simulink model "mppt"  (R2025b)
settings: Solver=VariableStepAuto  StartTime=0.0  StopTime=3  RelTol=1e-3
undefined symbols (not defined in the file): magnitude
libraries: spsParallelRLCBranchLib x8, spsVoltageMeasurementLib x3, spsCurrentMeasurementLib x2, spsDiodeLib x2, spsIGBTDiodeLib x2, spsPVArrayLib x2, eePwmGenerator x2, sps_lib x1, spspowerguiLib x1
settings Model: Creator=周宇轩  LastModifiedBy=yuxuan
settings SolverCC: ZeroCrossAlgorithm=Adaptive
settings DataIOCC: Refine=10
settings DebuggingCC: MaskedZcDiagnostic=none  IgnoredZcDiagnostic=none
settings RTWCC: GPUComputeCapability=3.5

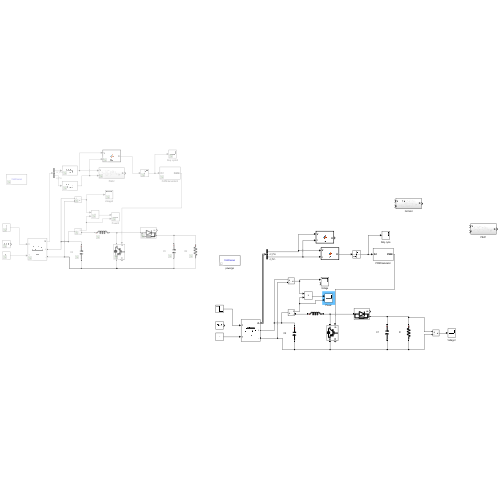
[thumbnail: Simulink's stored preview of the top-level diagram]
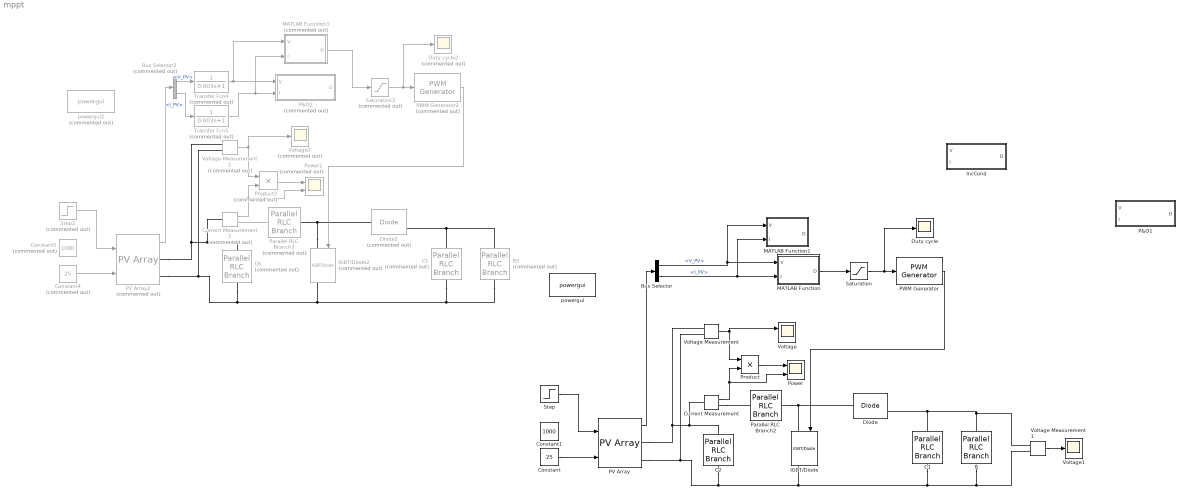
== system mppt ==
  Bus Selector : BusSelector  OutputSignals=V_PV,I_PV
  Bus Selector2 : BusSelector  Commented=on  OutputSignals=V_PV,I_PV
  C1 : spsParallelRLCBranchLib/Parallel RLC Branch  LConnTagsString=a  RConnTagsString=__new0  BranchType=C  Resistance=0  Inductance=0  SetiL0=off  InitialCurrent=0  Capacitance=1e-3  Setx0=off  InitialVoltage=0  Measurements=None
  C2 : spsParallelRLCBranchLib/Parallel RLC Branch  LConnTagsString=a  RConnTagsString=__new0  BranchType=C  Resistance=0  Inductance=0  SetiL0=off  InitialCurrent=0  Capacitance=2e-3  Setx0=off  InitialVoltage=0  Measurements=None
  C5 : spsParallelRLCBranchLib/Parallel RLC Branch  Commented=on  LConnTagsString=a  RConnTagsString=__new0  BranchType=C  Resistance=0  Inductance=0  SetiL0=off  InitialCurrent=0  Capacitance=1e-3  Setx0=off  InitialVoltage=0  Measurements=None
  C6 : spsParallelRLCBranchLib/Parallel RLC Branch  Commented=on  LConnTagsString=a  RConnTagsString=__new0  BranchType=C  Resistance=0  Inductance=0  SetiL0=off  InitialCurrent=0  Capacitance=1e-3  Setx0=off  InitialVoltage=0  Measurements=None
  Constant : Constant  Value=25
  Constant1 : Constant  Value=1000
  Constant4 : Constant  Commented=on  Value=25
  Constant5 : Constant  Commented=on  Value=1000
  Current Measurement : spsCurrentMeasurementLib/Current Measurement  PhasorSimulation=off  OutputType=Complex  PSBequivalent=0
  Current Measurement2 : spsCurrentMeasurementLib/Current Measurement  Commented=on  PhasorSimulation=off  OutputType=Complex  PSBequivalent=0
  Diode : spsDiodeLib/Diode  Ron=0.001  Lon=0  Vf=0.8  IC=0  UseSnubber=0  Rs=500  Cs=250e-9  Measurements=on
  Diode2 : spsDiodeLib/Diode  Commented=on  Ron=0.001  Lon=0  Vf=0.8  IC=0  UseSnubber=0  Rs=500  Cs=250e-9  Measurements=on
  Duty cycle : Scope
      settings: ActiveDisplayYMinimum=-0.03987  ActiveDisplayYMaximum=0.35887
  Duty cycle2 : Scope  Commented=on
      settings: ActiveDisplayYMinimum=-0.03987  ActiveDisplayYMaximum=0.35887  DataLoggingVariableName=ScopeData4
  IGBT/Diode : spsIGBTDiodeLib/IGBT//Diode  Ron=1e-3  Rs=1e5  Cs=inf  Measurements=on
  IGBT/Diode2 : spsIGBTDiodeLib/IGBT//Diode  Commented=on  Ron=1e-3  Rs=1e5  Cs=inf  Measurements=on
  IncCond : Subsystem
  MATLAB Function : MATLAB Function  TreatAsAtomicUnit=on
  MATLAB Function1 : MATLAB Function  TreatAsAtomicUnit=on
  MATLAB Function3 : MATLAB Function  Commented=on  TreatAsAtomicUnit=on
  P&O1 : Subsystem
  P&O2 : Subsystem  Commented=on
  PV Array : spsPVArrayLib/PV Array  Npar=40  Nser=10  PlotType=array @ 25 deg.C & specified irradiances  S_vec="[ 1000  600  100 ]"  Temp_C_vec="[ 45 25  ]"  ModuleName=User-defined  PlotWhenSelected=off  Pm=213.15  Ncell=60  Voc=36.3  Isc=7.84  Vm=29  Im=7.35  beta_Voc_pc=-0.36099  alpha_Isc_pc=0.102  beta_Voc=-0.13104  alpha_Isc=0.0079968  IL=7.8654  I0=2.9273e-10  nI=0.98119  Rsh=313.0553  Rs=0.39381  RobustModel=off  RobustCellTemperature=313.3991  BAL=on  Tc=1e-6  Tfilter=5e-5
  PV Array2 : spsPVArrayLib/PV Array  Commented=on  Npar=40  Nser=10  PlotType=array @ 25 deg.C & specified irradiances  S_vec="[ 1000  600  100 ]"  Temp_C_vec="[ 45 25  ]"  ModuleName=User-defined  PlotWhenSelected=off  Pm=213.15  Ncell=60  Voc=36.3  Isc=7.84  Vm=29  Im=7.35  beta_Voc_pc=-0.36099  alpha_Isc_pc=0.102  beta_Voc=-0.13104  alpha_Isc=0.0079968  IL=7.8654  I0=2.9273e-10  nI=0.98119  Rsh=313.0553  Rs=0.39381  RobustModel=off  RobustCellTemperature=313.3991  BAL=on  Tc=1e-6  Tfilter=5e-5
  PWM Generator : eePwmGenerator/PWM Generator  CarrCount=Up  Tper=0.0001  Tdelay=0  Ts=5e-6
  PWM Generator2 : eePwmGenerator/PWM Generator  Commented=on  CarrCount=Up  Tper=0.001  Tdelay=0  Ts=5e-5
  Parallel RLC Branch2 : spsParallelRLCBranchLib/Parallel RLC Branch  LConnTagsString=a  RConnTagsString=__new0  BranchType=L  Resistance=0  Inductance=3e-3  SetiL0=off  InitialCurrent=0  Capacitance=0  Setx0=off  InitialVoltage=0  Measurements=None
  Parallel RLC Branch3 : spsParallelRLCBranchLib/Parallel RLC Branch  Commented=on  LConnTagsString=a  RConnTagsString=__new0  BranchType=L  Resistance=0  Inductance=1e-3  SetiL0=off  InitialCurrent=0  Capacitance=0  Setx0=off  InitialVoltage=0  Measurements=None
  Power : Scope  NumInputPorts=2
      settings: ActiveDisplayYMinimum=-12032.8561078076  ActiveDisplayYMaximum=108295.70497026842
  Power2 : Scope  Commented=on  NumInputPorts=2
      settings: ActiveDisplayYMinimum=12927.91073  ActiveDisplayYMaximum=92933.50391  DataLoggingVariableName=ScopeData5
  Product : Product
  Product2 : Product  Commented=on
  R : spsParallelRLCBranchLib/Parallel RLC Branch  LConnTagsString=a  RConnTagsString=__new0  BranchType=R  Resistance=2  Inductance=0  SetiL0=off  InitialCurrent=0  Capacitance=0  Setx0=off  InitialVoltage=0  Measurements=None
  R2 : spsParallelRLCBranchLib/Parallel RLC Branch  Commented=on  LConnTagsString=a  RConnTagsString=__new0  BranchType=R  Resistance=2  Inductance=0  SetiL0=off  InitialCurrent=0  Capacitance=0  Setx0=off  InitialVoltage=0  Measurements=None
  Saturation : Saturate  UpperLimit=0.95  LowerLimit=0.05
  Saturation2 : Saturate  Commented=on  UpperLimit=0.95  LowerLimit=0.05
  Step : Step  Time=0.5  Before=1e3  After=600  SampleTime=0
  Step2 : Step  Commented=on  Time=0.5  Before=1e3  After=600  SampleTime=0
  Transfer Fcn4 : TransferFcn  Commented=on  Denominator=[0.003 1]
  Transfer Fcn5 : TransferFcn  Commented=on  Denominator=[0.003 1]
  Voltage : Scope  NumInputPorts=2
      settings: MaximizeAxes=On  ActiveDisplayYMinimum=-41.254198006758806  ActiveDisplayYMaximum=371.28778206082933
  Voltage Measurement : spsVoltageMeasurementLib/Voltage Measurement  PhasorSimulation=off  OutputType=Complex  PSBequivalent=0
  Voltage Measurement1 : spsVoltageMeasurementLib/Voltage Measurement  PhasorSimulation=off  OutputType=Complex  PSBequivalent=0
  Voltage Measurement2 : spsVoltageMeasurementLib/Voltage Measurement  Commented=on  PhasorSimulation=off  OutputType=Complex  PSBequivalent=0
  Voltage1 : Scope
      settings: MaximizeAxes=On  ActiveDisplayYMinimum=-41.254198006758806  ActiveDisplayYMaximum=371.28778206082933  DataLoggingVariableName=ScopeData2
  Voltage2 : Scope  Commented=on
      settings: MaximizeAxes=On  ActiveDisplayYMinimum=-213.56323  ActiveDisplayYMaximum=413.80386  DataLoggingVariableName=ScopeData6
  powergui : sps_lib/powergui  Priority=1  SimulationMode=Continuous  SampleTime=50e-6  frequency=60  Iterations=50  frequencyindice=0  Pbase=100e6  ErrMax=1e-4  UnitsV=kV  UnitsW=MW  buscounter=0  FunctionMessages=off  echomessages=off  EnableUseOfTLC=off  CurrentSourceSwitches=off  DisableSnubberDevices=off  DisableRonSwitches=off  DisableVfSwitches=off  DisplayEquations=off  AutomaticDiscreteSolvers=off  SolverType=Tustin/Backward Euler (TBE)  Interpol=off  ExternalGateDelay=off  methode=off  Ts=100  x0status=blocks  SPID=on  SwTol=0  HookPort=off  NonlinearTolerance=1e-4  nMaxIteration=100  ContinueOnMaxIteration=off  RestoreLinks=warning  ResistiveCurrentMeasurement=off  Frange=[0:2:500]  Ylog=off  Xlog=on  ShowGrid=off  save=off  variable=ZData  structure=0  ZoomFFT=off  StartTime=0.0  cycles=1  DisplayStyle=1  fundamental=60  FreqAxis=off  MaxFrequency=1000  frequencyindicesteady=1  RmsSteady=1  display=off
  powergui2 : spspowerguiLib/powergui  Priority=1  Commented=on  SimulationMode=Continuous  SampleTime=50e-6  frequency=60  Iterations=50  frequencyindice=0  Pbase=100e6  ErrMax=1e-4  UnitsV=kV  UnitsW=MW  buscounter=0  FunctionMessages=off  echomessages=off  EnableUseOfTLC=off  CurrentSourceSwitches=off  DisableSnubberDevices=off  DisableRonSwitches=off  DisableVfSwitches=off  DisplayEquations=off  AutomaticDiscreteSolvers=off  SolverType=Tustin/Backward Euler (TBE)  Interpol=off  ExternalGateDelay=off  methode=off  Ts=100  x0status=blocks  SPID=on  SwTol=0  HookPort=off  NonlinearTolerance=1e-4  nMaxIteration=100  ContinueOnMaxIteration=off  RestoreLinks=warning  ResistiveCurrentMeasurement=off  Frange=[0:2:500]  Ylog=off  Xlog=on  ShowGrid=off  save=off  variable=ZData  structure=0  ZoomFFT=off  StartTime=0.0  cycles=1  DisplayStyle=1  fundamental=60  FreqAxis=off  MaxFrequency=1000  frequencyindicesteady=1  RmsSteady=1  display=off
  wires:
  Constant/1 -> PV Array/2
  Bus Selector/1 -> MATLAB Function1/1(V), MATLAB Function/1(V)  "<V_PV>"
  Bus Selector/2 -> MATLAB Function1/2(I), MATLAB Function/2(I)  "<I_PV>"
  PV Array/1 -> Bus Selector/1
  Current Measurement/1 -> Power/2, Product/2
  Product/1 -> Power/1
  Voltage Measurement/1 -> Voltage/1, Product/1
  PWM Generator/1 -> IGBT/Diode/1
  Saturation/1 -> Duty cycle/1, PWM Generator/1
  Current Measurement2/1 -> Power2/2, Product2/2
  Saturation2/1 -> Duty cycle2/1, PWM Generator2/1
  Product2/1 -> Power2/1
  MATLAB Function3/1(D) -> Saturation2/1
  Voltage Measurement2/1 -> Voltage2/1, Product2/1
  PWM Generator2/1 -> IGBT/Diode2/1
  Constant4/1 -> PV Array2/2
  Bus Selector2/1 -> Transfer Fcn4/1  "<V_PV>"
  Bus Selector2/2 -> Transfer Fcn5/1  "<I_PV>"
  Step2/1 -> PV Array2/1
  Transfer Fcn4/1 -> P&O2/1(V), MATLAB Function3/1(V)
  Transfer Fcn5/1 -> P&O2/2(I), MATLAB Function3/2(I)
  PV Array2/1 -> Bus Selector2/1
  Step/1 -> PV Array/1
  MATLAB Function/1(D) -> Saturation/1
  Voltage Measurement1/1 -> Voltage1/1
  connections:
  Diode/LConn1 -- Parallel RLC Branch2/RConn1 -- IGBT/Diode/LConn1
  PV Array/RConn2 -- Voltage Measurement/LConn2 -- R/RConn1 -- Voltage Measurement1/LConn2 -- C1/RConn1 -- IGBT/Diode/RConn1 -- C2/RConn1
  R/LConn1 -- Voltage Measurement1/LConn1 -- C1/LConn1 -- Diode/RConn1
  PV Array/RConn1 -- Voltage Measurement/LConn1 -- Current Measurement/LConn1 -- C2/LConn1
  Current Measurement/RConn1 -- Parallel RLC Branch2/LConn1
  IGBT/Diode2/RConn1 -- PV Array2/RConn2 -- Voltage Measurement2/LConn2 -- C6/RConn1 -- R2/RConn1 -- C5/RConn1
  C6/LConn1 -- PV Array2/RConn1 -- Voltage Measurement2/LConn1 -- Current Measurement2/LConn1
  Diode2/RConn1 -- R2/LConn1 -- C5/LConn1
  IGBT/Diode2/LConn1 -- Diode2/LConn1 -- Parallel RLC Branch3/RConn1
  Current Measurement2/RConn1 -- Parallel RLC Branch3/LConn1

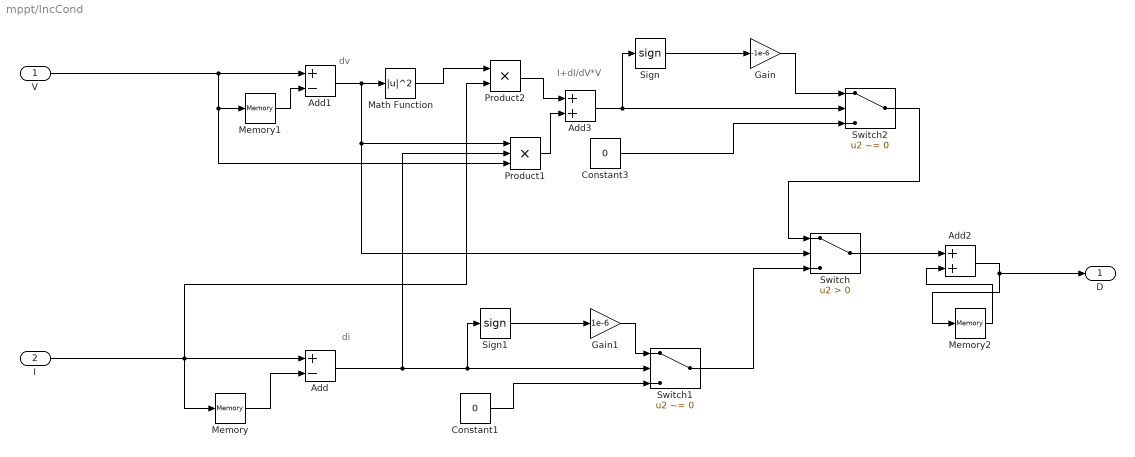
== system mppt/IncCond ==
  note: I+dI/dV*V
  note: di
  note: dv
  V : Inport
  I : Inport  Port=2
  Add : Sum  Inputs=+-
  Add1 : Sum  Inputs=+-
  Add2 : Sum
  Add3 : Sum
  Constant1 : Constant  Value=0
  Constant3 : Constant  Value=0
  Gain : Gain  Gain=-1e-6
  Gain1 : Gain  Gain=1e-6
  Math Function : Math  Operator=magnitude^2
  Memory : Memory
  Memory1 : Memory
  Memory2 : Memory
  Product1 : Product  Inputs=3
  Product2 : Product
  Sign : Signum
  Sign1 : Signum
  Switch : Switch  Criteria=u2 > Threshold  SaturateOnIntegerOverflow=off  InputSameDT=off
  Switch1 : Switch  Criteria=u2 ~= 0  SaturateOnIntegerOverflow=off  InputSameDT=off
  Switch2 : Switch  Criteria=u2 ~= 0  SaturateOnIntegerOverflow=off  InputSameDT=off
  D : Outport
  wires:
  Memory/1 -> Add/2
  V/1 -> Product1/3, Memory1/1, Add1/1
  Add1/1 -> Switch/2, Product1/1, Math Function/1
  Memory1/1 -> Add1/2
  I/1 -> Product2/2, Memory/1, Add/1
  Math Function/1 -> Product2/1
  Product2/1 -> Add3/1
  Product1/1 -> Add3/2
  Add3/1 -> Sign/1, Switch2/2
  Constant3/1 -> Switch2/3
  Gain/1 -> Switch2/1
  Switch2/1 -> Switch/1
  Constant1/1 -> Switch1/3
  Add/1 -> Product1/2, Sign1/1, Switch1/2
  Gain1/1 -> Switch1/1
  Switch1/1 -> Switch/3
  Switch/1 -> Add2/1
  Add2/1 -> Memory2/1, D/1
  Memory2/1 -> Add2/2
  Sign1/1 -> Gain1/1
  Sign/1 -> Gain/1

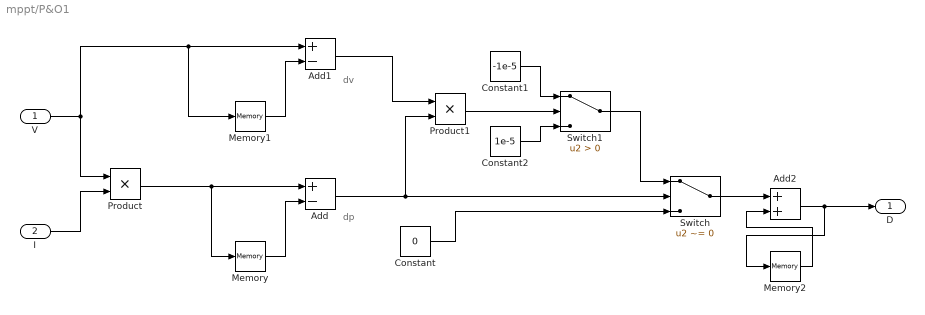
== system mppt/P&O1 ==
  note: dp
  note: dv
  V : Inport
  I : Inport  Port=2
  Add : Sum  Inputs=+-
  Add1 : Sum  Inputs=+-
  Add2 : Sum
  Constant : Constant  Value=0
  Constant1 : Constant  Value=-1e-5
  Constant2 : Constant  Value=1e-5
  Memory : Memory
  Memory1 : Memory
  Memory2 : Memory  InitialCondition=0.7
  Product : Product
  Product1 : Product
  Switch : Switch  Criteria=u2 ~= 0  SaturateOnIntegerOverflow=off  InputSameDT=off
  Switch1 : Switch  Criteria=u2 > Threshold  SaturateOnIntegerOverflow=off  InputSameDT=off
  D : Outport
  wires:
  I/1 -> Product/2
  Product/1 -> Memory/1, Add/1
  Memory/1 -> Add/2
  Add/1 -> Product1/2, Switch/2
  Constant/1 -> Switch/3
  V/1 -> Product/1, Add1/1, Memory1/1
  Add1/1 -> Product1/1
  Memory1/1 -> Add1/2
  Product1/1 -> Switch1/2
  Constant1/1 -> Switch1/1
  Constant2/1 -> Switch1/3
  Switch1/1 -> Switch/1
  Switch/1 -> Add2/1
  Memory2/1 -> Add2/2
  Add2/1 -> D/1, Memory2/1

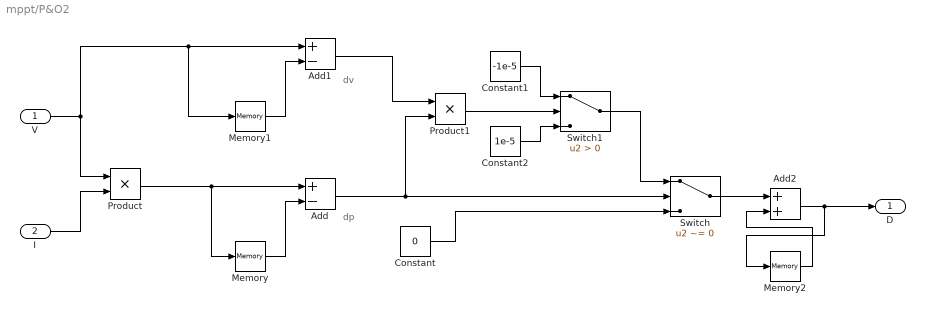
== system mppt/P&O2 ==
  note: dp
  note: dv
  V : Inport
  I : Inport  Port=2
  Add : Sum  Inputs=+-
  Add1 : Sum  Inputs=+-
  Add2 : Sum
  Constant : Constant  Value=0
  Constant1 : Constant  Value=-1e-5
  Constant2 : Constant  Value=1e-5
  Memory : Memory
  Memory1 : Memory
  Memory2 : Memory  InitialCondition=0.7
  Product : Product
  Product1 : Product
  Switch : Switch  Criteria=u2 ~= 0  SaturateOnIntegerOverflow=off  InputSameDT=off
  Switch1 : Switch  Criteria=u2 > Threshold  SaturateOnIntegerOverflow=off  InputSameDT=off
  D : Outport
  wires:
  I/1 -> Product/2
  Product/1 -> Memory/1, Add/1
  Memory/1 -> Add/2
  Add/1 -> Product1/2, Switch/2
  Constant/1 -> Switch/3
  V/1 -> Product/1, Add1/1, Memory1/1
  Add1/1 -> Product1/1
  Memory1/1 -> Add1/2
  Product1/1 -> Switch1/2
  Constant1/1 -> Switch1/1
  Constant2/1 -> Switch1/3
  Switch1/1 -> Switch/1
  Switch/1 -> Add2/1
  Memory2/1 -> Add2/2
  Add2/1 -> D/1, Memory2/1

== matlab function mppt/MATLAB Function ==
  settings: updateMethod=DISCRETE
  data: V input; D output; I input
function D = PO(V, I)
% Direct-duty P&O MPPT for Boost converter
%
% PWM sample time = 5e-6 s
% N = 1000 -> MPPT update period = 5e-3 s
% 每50个PWM周期更新一次MPPT

persistent Dprev Pprev direction
persistent sumP sampleCount initialized

%% Parameters
Dinit = 0.30;
Dmin  = 0.05;
Dmax  = 0.90;

N = 1000;                 % 1000*5e-6 = 5 ms

deltaD_track = 5e-4;      % 寻优时使用
deltaD_steady = 5e-5;     % MPP附近使用
Pdead = 100;              % 功率死区，单位 W

%% Initialization
if isempty(initialized)
    Dprev = Dinit;
    Pprev = 0;
    direction = 1;

    sumP = 0;
    sampleCount = 0;
    initialized = false;
end

%% Average instantaneous power
sumP = sumP + V*I;
sampleCount = sampleCount + 1;

% 两次MPPT更新之间保持D不变
D = Dprev;

if sampleCount < N
    return;
end

Pavg = sumP/N;

sumP = 0;
sampleCount = 0;

%% First measurement
if ~initialized
    Pprev = Pavg;
    initialized = true;

    % 第一次主动扰动
    Dnew = Dprev + direction*deltaD_track;
else
    dP = Pavg - Pprev;

    if dP > Pdead
        % 上一次扰动使功率增加，继续原方向
        step = deltaD_track;

    elseif dP < -Pdead
        % 上一次扰动使功率下降，反转方向
        direction = -direction;
        step = deltaD_track;

    else
        % 已接近MPP，只做很小的往返扰动
        direction = -direction;
        step = deltaD_steady;
    end

    Dnew = Dprev + direction*step;
    Pprev = Pavg;
end

%% Duty-cycle limitation
if Dnew >= Dmax
    Dnew = Dmax;
    direction = -1;

elseif Dnew <= Dmin
    Dnew = Dmin;
    direction = 1;
end

D = Dnew;
Dprev = Dnew;

end

== matlab function mppt/MATLAB Function3 ==
  settings: updateMethod=DISCRETE
  data: V input; D output; I input
function D = INC(V, I)

persistent Irev Vrev Drev
if isempty(Irev)
    Drev = 0.3;   % Initial duty cycle
    Vrev = 0;     % Previous voltage
    Irev = 0;     % Previous current
end

deltaD = 1e-6;   % Step size of duty cycle adjustment
dI = I - Irev;   % Change in current
dV = V - Vrev;   % Change in voltage

if dV ~= 0
    % Incremental Conductance condition: dI/dV ≈ -I/V
    if I + dI/dV * V ~= 0
        if I + dI/dV * V > 0
            D = Drev - deltaD;   % Left of MPP -> increase voltage (decrease duty)
        else
            D = Drev + deltaD;   % Right of MPP -> decrease voltage (increase duty)
        end
    else
        D = Drev;  % At MPP -> keep duty cycle unchanged
    end
else
    % If voltage is unchanged, use current variation
    if dI ~= 0
        if dI > 0
            D = Drev + deltaD;   % Current rising -> increase duty
        else
            D = Drev - deltaD;   % Current falling -> decrease duty
        end
    else
        D = Drev;  % No change -> keep duty cycle
    end
end

% Update stored values
Drev = D;
Vrev = V;
Irev = I;

end

== matlab function mppt/MATLAB Function1 ==
  settings: updateMethod=DISCRETE
  data: V input; D output; I input
function D = INC(V, I)
% Incremental Conductance MPPT for Boost converter
% 建议以固定离散周期调用，例如 Ts_mppt = 1e-3 s

persistent Vprev Iprev Dprev initialized

% Parameters
Dinit  = 0.30;
Dmin   = 0.05;
Dmax   = 0.90;

deltaD = 2e-4;    % 每次MPPT更新的占空比步长
epsV   = 0.10;    % 电压变化死区，单位 V
epsI   = 0.02;    % 电流变化死区，单位 A
epsG   = 1e-3;    % 增量电导判断死区，单位 A/V

if isempty(initialized)
    Dprev = Dinit;
    Vprev = V;
    Iprev = I;
    initialized = true;

    D = Dprev;
    return;
end

dV = V - Vprev;
dI = I - Iprev;

D = Dprev;

if abs(dV) <= epsV
    % 电压基本不变
    if abs(dI) <= epsI
        % 电压、电流均基本不变，保持占空比
        D = Dprev;

    elseif dI > 0
        % 位于MPP左侧：需要提高PV电压
        % Boost中提高PV电压 -> 减小占空比
        D = Dprev - deltaD;

    else
        % 位于MPP右侧：需要降低PV电压
        % Boost中降低PV电压 -> 增大占空比
        D = Dprev + deltaD;
    end

else
    % dP/dV = I + V*dI/dV
    conductanceError = dI/dV + I/max(abs(V), 1);

    if abs(conductanceError) <= epsG
        % 接近MPP，保持占空比
        D = Dprev;

    elseif conductanceError > 0
        % dP/dV > 0，位于MPP左侧，需要提高PV电压
        D = Dprev - deltaD;

    else
        % dP/dV < 0，位于MPP右侧，需要降低PV电压
        D = Dprev + deltaD;
    end
end

% Duty-cycle limitation
D = min(max(D, Dmin), Dmax);

% Update stored values
Dprev = D;
Vprev = V;
Iprev = I;

end
